simulink model "simulink_2009a_model"  (Simulink 7.3)
settings: Solver=ode15s  StartTime=0.0  StopTime=10  RelTol=1e-3
libraries: simulink x1
settings Model: Creator=osabio  LastModifiedBy=osabio
settings DataIOCC: ReturnWorkspaceOutputs=off
settings DebuggingCC: FcnCallInpInsideContextMsg=Enable All  StrictBusMsg=ErrorLevel1

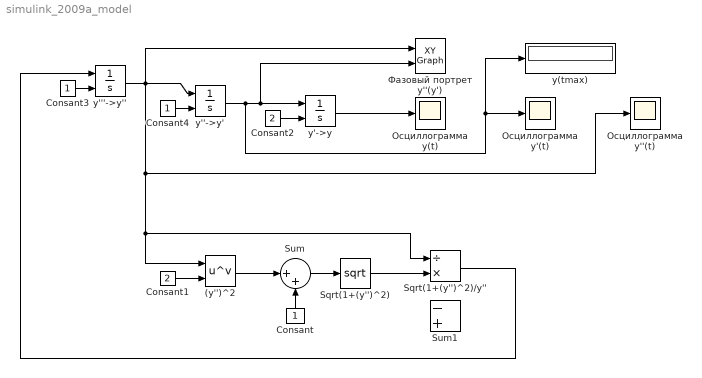
== system simulink_2009a_model ==
  (y'')^2 : Math  Operator=pow  SaturateOnIntegerOverflow=on
  Consant : Constant
  Consant1 : Constant  Value=2
  Consant2 : Constant  Value=2
  Consant3 : Constant
  Consant4 : Constant
  Sqrt(1+(y'')^2) : Math  Operator=sqrt  SaturateOnIntegerOverflow=on
  Sqrt(1+(y'')^2)/y'' : Product  Inputs=/*
  Sum : Sum  Inputs=|++
  Sum1 : Sum  Inputs=-+
      settings: AttributesFormatString=Sqrt(1+(y'')^2)-y''
  y'''->y'' : Integrator  InitialConditionSource=external
  y''->y' : Integrator  InitialConditionSource=external
  y'->y : Integrator  InitialConditionSource=external
  y(tmax) : Display
  Осциллограмма y''(t) : Scope
      settings: SaveName=ScopeData2
  Осциллограмма y'(t) : Scope
  Осциллограмма y(t) : Scope
  Фазовый портрет y''(y') : simulink/Sinks/XY Graph  xmin=0  xmax=20  ymin=0  ymax=70  st=-1
  wires:
  y'''->y''/1 -> y''->y'/1, Фазовый портрет y''(y')/1, (y'')^2/1, Sqrt(1+(y'')^2)/y''/1, Осциллограмма y''(t)/1
  y''->y'/1 -> y'->y/1, Фазовый портрет y''(y')/2, Осциллограмма y'(t)/1, y(tmax)/1
  Consant/1 -> Sum/2
  Consant1/1 -> (y'')^2/2
  (y'')^2/1 -> Sum/1
  Sum/1 -> Sqrt(1+(y'')^2)/1
  Consant2/1 -> y'->y/2
  Consant4/1 -> y''->y'/2
  Consant3/1 -> y'''->y''/2
  y'->y/1 -> Осциллограмма y(t)/1
  Sqrt(1+(y'')^2)/y''/1 -> y'''->y''/1
  Sqrt(1+(y'')^2)/1 -> Sqrt(1+(y'')^2)/y''/2
